simulink model "test_delfttyre_cpi2"  (Simulink 6.4)
settings: Solver=ode45  SolverMode=SingleTasking  StartTime=0.0  StopTime=2*pi  FixedStep=0.02  MaxStep=0.01  RelTol=1e-5  AbsTol=1e-5
libraries: Delft_Tyre_dtlib x1, simulink x1, Delft_Tyre_sm1glib x1
settings Model: Creator=hofstadrhmtvd  LastModifiedBy=hofstadrhmtvd  ExtModeTrigMode=oneshot  ExtModeArmWhenConnect=off
settings SolverCC: InitialStep=0.001
settings DataIOCC: LimitDataPoints=off  SignalLoggingName=sigsOut
settings OptimizationCC: BooleanDataType=off
settings DebuggingCC: SolverPrmCheckMsg=none  StrictBusMsg=ErrorLevel1
settings HardwareCC: TargetHWDeviceType=32-bit Generic  TargetUnknown=on  ProdEqTarget=off

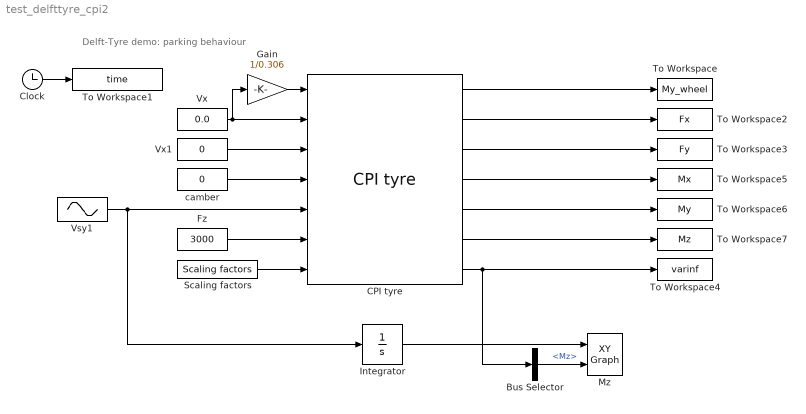
== system test_delfttyre_cpi2 ==
  note: Delft-Tyre demo: parking behaviour
  Bus Selector : BusSelector  OutputSignals=Mz
  CPI tyre : Delft_Tyre_dtlib/Simulink/CPI tyre  Tag=CPI tyre  SystemSampleTime=-1  idtyre=1  tpfname='TNO_car205_60R15.tir'  side_mode=(3xxx) symmetric  dyn_mode=(xx2x) relaxation behaviour - non-linear  mf_mode=(xxx5) combined+turnslip  use_mode=1e8  disp_debug=off
  Clock : Clock
      settings: Decimation=10
  Fz : Constant  Value=3000  OutDataType=fixdt(1,16,0)  ConRadixGroup=Use specified scaling  OutScaling=[]  SampleTime=inf  FramePeriod=inf
  Gain : Gain  Gain=1/0.306  ParameterDataType=fixdt(1,16,0)  ParameterScaling=[]  OutDataType=fixdt(1,16,0)  OutScaling=[]  SaturateOnIntegerOverflow=on
  Integrator : Integrator
  Mz : simulink/Sinks/XY Graph  SystemSampleTime=-1  xmin=-0.3  xmax=0.3  ymin=-250  ymax=250  st=-1
  Scaling factors : Delft_Tyre_sm1glib/SimMechanics 1G/Scaling factors  Tag=Scaling factors  SystemSampleTime=-1  LMUX=1  LKX=1  LMUY=1  LKY=1  LKYC=1  LTR=1  LKZC=1
  To Workspace : ToWorkspace  VariableName=My_wheel  SampleTime=-1  SaveFormat=Array
  To Workspace1 : ToWorkspace  VariableName=time  SampleTime=-1  SaveFormat=Array
  To Workspace2 : ToWorkspace  VariableName=Fx  SampleTime=-1  SaveFormat=Array
  To Workspace3 : ToWorkspace  VariableName=Fy  SampleTime=-1  SaveFormat=Array
  To Workspace4 : ToWorkspace  VariableName=varinf  SampleTime=-1  SaveFormat=Array
  To Workspace5 : ToWorkspace  VariableName=Mx  SampleTime=-1  SaveFormat=Array
  To Workspace6 : ToWorkspace  VariableName=My  SampleTime=-1  SaveFormat=Array
  To Workspace7 : ToWorkspace  VariableName=Mz  SampleTime=-1  SaveFormat=Array
  Vsy1 : Sin  Amplitude=0.3  Phase=pi/2  SampleTime=0
  Vx : Constant  Value=0.0  OutDataType=fixdt(1,16,0)  ConRadixGroup=Use specified scaling  OutScaling=[]  SampleTime=inf  FramePeriod=inf
  Vx1 : Constant  Value=0  OutDataType=fixdt(1,16,0)  ConRadixGroup=Use specified scaling  OutScaling=[]  SampleTime=inf  FramePeriod=inf
  camber : Constant  Value=0  OutDataType=fixdt(1,16,0)  ConRadixGroup=Use specified scaling  OutScaling=[]  SampleTime=inf  FramePeriod=inf
  wires:
  Clock/1 -> To Workspace1/1
  Scaling factors/1 -> CPI tyre/7
  Vx1/1 -> CPI tyre/3
  camber/1 -> CPI tyre/4
  Fz/1 -> CPI tyre/6
  CPI tyre/1 -> To Workspace/1
  CPI tyre/2 -> To Workspace2/1
  CPI tyre/3 -> To Workspace3/1
  CPI tyre/4 -> To Workspace5/1
  CPI tyre/6 -> To Workspace7/1
  CPI tyre/5 -> To Workspace6/1
  Vx/1 -> Gain/1, CPI tyre/2
  CPI tyre/7 -> To Workspace4/1, Bus Selector/1
  Vsy1/1 -> Integrator/1, CPI tyre/5
  Gain/1 -> CPI tyre/1
  Bus Selector/1 -> Mz/2  "<Mz>"
  Integrator/1 -> Mz/1
